simulink model "Combined_DCconv_andMPPT"  (R2023a)
settings: Solver=ode23s  StartTime=0.0  StopTime=0.1  MaxStep=0.0000001  RelTol=1e-4  AbsTol=1e-4
values from neighbouring files (symbols this model uses):
  A = Aoff    [BoostConverterHybrid.m]    (also in PV_Params.mat = 1.3)
  C = [0 1]    [BoostConverterHybrid.m]    (also in boost_converter_sfcnv3.m = u(4); params_dcdc.m = 0.00012878; params_forEVcharge.m = 0.00010675)
  E = u(1)    [boost_converter_sfcnv3.m]    (also in params_forEVcharge.m = 90)
  Isc = 8.61    [PV_Params.mat]    (also in parameterEstimationv2.m = 5.45)
  Ki = 0.05    [PV_Params.mat]
  Kv = -0.32    [PV_Params.mat]
  L = 1    [BoostConverterHybrid.m]    (also in boost_converter_sfcnv3.m = u(3); params_dcdc.m = 0.00035; params_forEVcharge.m = 0.008945)
  Ns = 60    [PV_Params.mat]
  R = 1    [BoostConverterHybrid.m]    (also in boost_converter_sfcnv3.m = u(5); params_dcdc.m = 4.6; params_forEVcharge.m = 48.48)
  Rp = 415    [PV_Params.mat]    (also in battery_params_v2.m = 0.003103; parameterEstimationv2.m = R_p)
  Rs = 0.22    [PV_Params.mat]    (also in battery_params_v2.m = 0.010822; parameterEstimationv2.m = R_s)
  T = 298    [parameterEstimationv2.m]    (also in params_dcdc.m = 1e-05; params_forEVcharge.m = 1e-05)
  Voc = 38.41    [PV_Params.mat]    (also in parameterEstimationv2.m = 43.6)
undefined symbols (not defined in the file or in its folder): sigbuilder_block
libraries: simulink x2, slpidlib x1, SignalEditorBlockLib x1
settings Model: Creator=gabrielcrisan  LastModifiedBy=gabrielcrisan

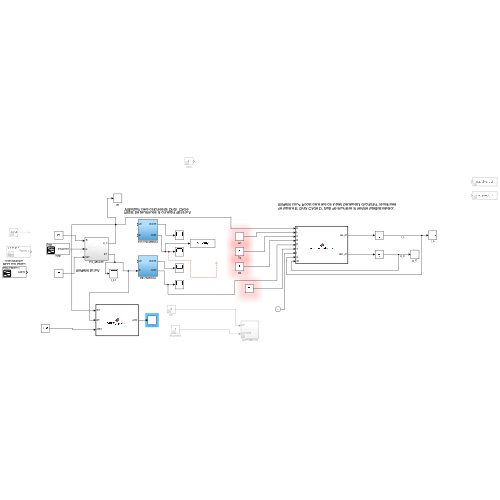
[thumbnail: Simulink's stored preview of the top-level diagram]
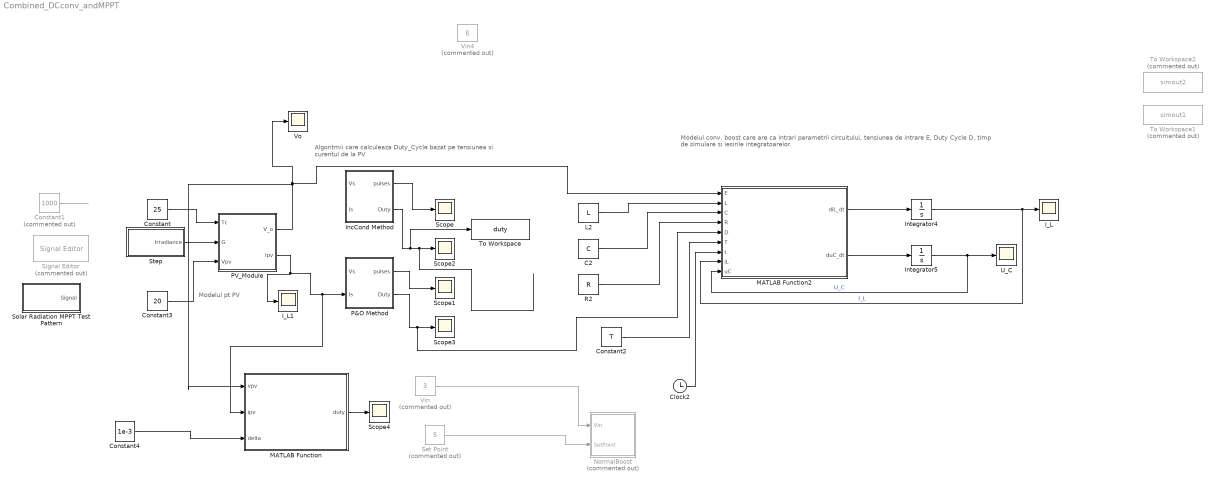
== system Combined_DCconv_andMPPT ==
  note: Modelul pt PV
  note: Algoritmii care calculeaza Duty_Cycle bazat pe tensiunea si curentul de la PV
  note: Modelul conv. boost care are ca intrari parametrii circuitului, tensiunea de intrare E, Duty Cycle D, timp de simulare si iesirile integratoarelor.
  C2 : Constant  Value=C
  Clock2 : Clock
  Constant : Constant  Value=25
  Constant1 : Constant  Commented=on  Value=1000
  Constant2 : Constant  Value=T
  Constant3 : Constant  Value=20
  Constant4 : Constant  Value=1e-3
  I_L : Scope
  I_L1 : Scope
  IncCond Method : Subsystem  VariantControl=MPPT_IncCond
  Integrator4 : Integrator
  Integrator5 : Integrator
  L2 : Constant  Value=L
  MATLAB Function : MATLAB Function  TreatAsAtomicUnit=on
  MATLAB Function2 : MATLAB Function  TreatAsAtomicUnit=on
  NormalBoost : Subsystem  Commented=on
  P&O Method : Subsystem  VariantControl=MPPT_PandO
  PV_Module : Subsystem
  R2 : Constant  Value=R
  Scope{,1..4} (5 alike) : Scope
  Set Point : Constant  Commented=on  Value=5
  Signal Editor : SignalEditorBlockLib/Signal Editor  Commented=on  FileName=untitled.mat  ActiveScenario=Scenario  ActiveSignal=Signal 1  IsBus=off  OutputBusObjectStr=Bus: BusObject  SampleTime=0  Interpolate=off  ZeroCross=off  OutputAfterFinalValue=Setting to zero  Unit=inherit  PreserveSignalName=on  ApplySigPropsToAllScenarios=on
  Solar Radiation MPPT Test Pattern : Subsystem  Tag=STV Subsys  LoadFcn=sigbuilder_block('load',[1935 57 649 359 ]);  StartFcn=sigbuilder_block('start');  StopFcn=sigbuilder_block('stop');  ClipboardFcn=sigbuilder_block('clipboard');  mask(Sigbuilder block){tuvar=[0:10]}
      mask help: Simulink:masks:SigbuilderBlock_MD
      mask init:
      | if ~strcmp(get_param(bdroot(gcbh),'SimulationStatus'),'stopped') tuvar = sigbuilder_block('maskInit'); end
      settings: CopyFcn=sigbuilder_block('copy');  DeleteFcn=sigbuilder_block('delete');  ModelCloseFcn=sigbuilder_block('modelClose');  PreSaveFcn=sigbuilder_block('preSave');  PauseFcn=sigbuilder_block('pause');  ContinueFcn=sigbuilder_block('continue');  NameChangeFcn=sigbuilder_block('namechange');  OpenFcn=sigbuilder_block('open',[330.75 60 648.75 359.25 ]);  CloseFcn=sigbuilder_block('close');
      mask Display: plot(0, 0, 100, 100,[2, 2, 32, 32, 2], [68, 8, 8, 68, 68],[32, 2], [38, 38], [32, 19, 2],[53, 60, 44], [32, 17, 17, 2],[16, 16, 31, 31]);txt = getActiveGroup(gcbh);text(2, 100, txt,'verticalAlignment', 'top');
  Step : Subsystem  Tag=STV Subsys  LoadFcn=sigbuilder_block('load');  StartFcn=sigbuilder_block('start');  StopFcn=sigbuilder_block('stop');  ClipboardFcn=sigbuilder_block('clipboard');  VariantControl=Step  mask(Sigbuilder block){tuvar=[0:10]}
      mask help: Simulink:masks:SigbuilderBlock_MD
      mask init:
      | if ~strcmp(get_param(bdroot(gcbh),'SimulationStatus'),'stopped') tuvar = sigbuilder_block('maskInit'); end
      settings: CopyFcn=sigbuilder_block('copy');  DeleteFcn=sigbuilder_block('delete');  ModelCloseFcn=sigbuilder_block('modelClose');  PreSaveFcn=sigbuilder_block('preSave');  PauseFcn=sigbuilder_block('pause')  ContinueFcn=sigbuilder_block('continue')  NameChangeFcn=sigbuilder_block('namechange');  OpenFcn=sigbuilder_block('open',[1901 151 412 328 ]);  CloseFcn=sigbuilder_block('close');
      mask Display: plot(0, 0, 100, 100,[2, 2, 32, 32, 2], [68, 8, 8, 68, 68],[32, 2], [38, 38], [32, 19, 2],[53, 60, 44], [32, 17, 17, 2],[16, 16, 31, 31]);txt = getActiveGroup(gcbh);text(2, 100, txt,'verticalAlignment', 'top');
  To Workspace : ToWorkspace  VariableName=duty  SaveFormat=Timeseries  SampleTime=-1
  To Workspace1 : ToWorkspace  Commented=on  VariableName=simout1  SaveFormat=Timeseries  SampleTime=-1
  To Workspace2 : ToWorkspace  Commented=on  VariableName=simout2  SaveFormat=Timeseries  SampleTime=-1
  U_C : Scope
  Vin : Constant  Commented=on  Value=3
  Vin4 : Constant  Commented=on  Value=E
  Vo : Scope
  wires:
  C2/1 -> MATLAB Function2/3(C)
  Integrator4/1 -> MATLAB Function2/8(iL), I_L/1  "I_L"
  R2/1 -> MATLAB Function2/4(R)
  MATLAB Function2/1(diL_dt) -> Integrator4/1
  MATLAB Function2/2(duC_dt) -> Integrator5/1
  Clock2/1 -> MATLAB Function2/7(t)
  Constant2/1 -> MATLAB Function2/6(T)
  L2/1 -> MATLAB Function2/2(L)
  P&O Method/2(Duty) -> MATLAB Function2/5(D), Scope3/1
  Integrator5/1 -> U_C/1, MATLAB Function2/9(uC)  "U_C"
  IncCond Method/1(pulses) -> Scope/1
  P&O Method/1(pulses) -> Scope1/1
  IncCond Method/2(Duty) -> Scope2/1, To Workspace/1
  PV_Module/2(Ipv) -> MATLAB Function/2(ipv), P&O Method/2(Is), I_L1/1
  Constant1/1 -> ?
  Constant/1 -> PV_Module/1(Tc)
  PV_Module/1(V_o) -> MATLAB Function/1(vpv), Vo/1, MATLAB Function2/1(E)
  Constant3/1 -> PV_Module/3(Vpv)
  Step/1(Irradiance) -> PV_Module/2(G)
  Set Point/1 -> NormalBoost/2(SetPoint)
  Vin/1 -> NormalBoost/1(Vin)
  Constant4/1 -> MATLAB Function/3(delta)
  MATLAB Function/1(duty) -> Scope4/1

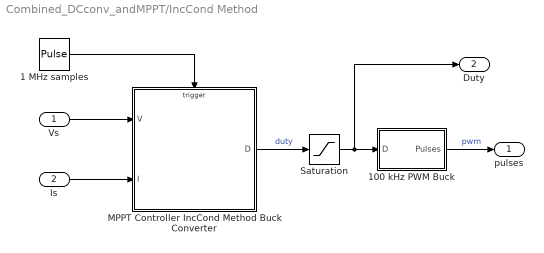
== system Combined_DCconv_andMPPT/IncCond Method ==
  Vs : Inport
  Is : Inport  Port=2
  1 MHz samples : DiscretePulseGenerator  PulseType=Time based  Period=0.000001  PulseWidth=5
  100 kHz PWM Buck : Subsystem  mask{Freq=100000}
      mask prompts: Freq "Frequency (Hz)"
  MPPT Controller IncCond Method Buck Converter : Stateflow chart  TreatAsAtomicUnit=on
  Saturation : Saturate  UpperLimit=1  LowerLimit=0  OutMin=[0]  OutMax=[1]
  pulses : Outport
  Duty : Outport  Port=2
  wires:
  Vs/1 -> MPPT Controller IncCond Method Buck Converter/1(V)
  MPPT Controller IncCond Method Buck Converter/1(D) -> Saturation/1  "duty"
  100 kHz PWM Buck/1(Pulses) -> pulses/1  "pwm"
  1 MHz samples/1 -> MPPT Controller IncCond Method Buck Converter/Trigger
  Saturation/1 -> Duty/1, 100 kHz PWM Buck/1(D)
  Is/1 -> MPPT Controller IncCond Method Buck Converter/2(I)

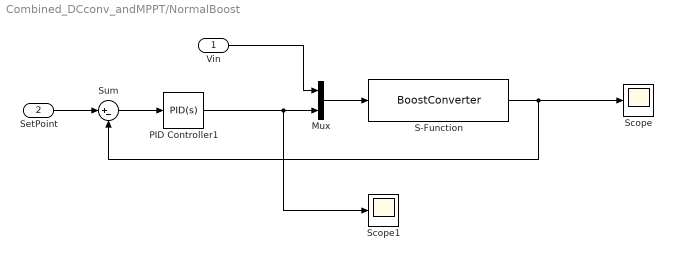
== system Combined_DCconv_andMPPT/NormalBoost ==
  Vin : Inport
  SetPoint : Inport  Port=2
  Mux : Mux  Inputs=2
  PID Controller1 : slpidlib/PID Controller  Controller=PID  Form=Parallel  TimeDomain=Continuous-time  UseExternalTs=off  SampleTime=-1  IntegratorMethod=Forward Euler  FilterMethod=Forward Euler  ControllerParametersSource=internal  P=10  I=0.2  UseKiTs=off  D=0  N=100  UseFilter=on  TunerSelectOption=Transfer Function Based (PID Tuner App)  InitialConditionSource=internal  InitialConditionForIntegrator=0  InitialConditionForFilter=0  DifferentiatorICPrevScaledInput=0  ExternalReset=none  TrackingMode=off  Kt=1  LimitOutput=off  SatLimitsSource=internal  UpperSaturationLimit=inf  LowerSaturationLimit=-inf  LinearizeAsGain=on  AntiWindupMode=none  Kb=1  LimitIntegrator=off  UpperIntegratorSaturationLimit=inf  LowerIntegratorSaturationLimit=-inf  POutMin=[]  POutMax=[]  IOutMin=[]  IOutMax=[]  DOutMin=[]  DOutMax=[]  NOutMin=[]  NOutMax=[]  SumOutMin=[]  SumOutMax=[]  SaturationOutMin=[]  SaturationOutMax=[]  PParamMin=[]  PParamMax=[]  IParamMin=[]  IParamMax=[]  DParamMin=[]  DParamMax=[]  NParamMin=[]  NParamMax=[]  KbParamMin=[]  KbParamMax=[]  KtParamMin=[]  KtParamMax=[]  KbOutMin=[]  KbOutMax=[]  KtOutMin=[]  KtOutMax=[]  IntegratorOutMin=[]  IntegratorOutMax=[]  FilterOutMin=[]  FilterOutMax=[]  SumI1OutMin=[]  SumI1OutMax=[]  SumI2OutMin=[]  SumI2OutMax=[]  SumI3OutMin=[]  SumI3OutMax=[]  SumI4OutMin=[]  SumI4OutMax=[]  SumDOutMin=[]  SumDOutMax=[]  DifferentiatorOutMin=[]  DifferentiatorOutMax=[]  FilterDiffOutCoefMin=[]  FilterDiffOutCoefMax=[]  ReciprocalOutMin=[]  ReciprocalOutMax=[]  SumDenOutMin=[]  SumDenOutMax=[]  SumNumOutMin=[]  SumNumOutMax=[]  DivideOutMin=[]  DivideOutMax=[]  UdiffTsProdOutMin=[]  UdiffTsProdOutMax=[]  NTsProdOutMin=[]  NTsProdOutMax=[]  UintegralTsProdOutMin=[]  UintegralTsProdOutMax=[]  UngainTsProdOutMin=[]  UngainTsProdOutMax=[]  ClampingZeroOutDataTypeStr=Inherit: Inherit via back propagation  ClampingZeroOutMin=[]  ClampingZeroOutMax=[]  FilterDenConstantOutDataTypeStr=Inherit: Inherit via back propagation  FilterDenConstantOutMin=[]  FilterDenConstantOutMax=[]  PCopyOutDataTypeStr=Inherit: Inherit via back propagation  PCopyOutMin=[]  PCopyOutMax=[]  NCopyOutDataTypeStr=Inherit: Inherit via back propagation  NCopyOutMin=[]  NCopyOutMax=[]  IntegratorContinuousStateAttributes=''  IntegratorStateMustResolveToSignalObject=off  IntegratorRTWStateStorageClass=Auto  FilterContinuousStateAttributes=''  FilterStateMustResolveToSignalObject=off  FilterRTWStateStorageClass=Auto  ParallelPVariant=InternalParameters  IdealPVariant=Disabled  IVariant=InternalParameters  DVariant=InternalParameters  IntegratorVariant=Continuous  SatVariant=Disabled  AWVariant=Passthrough  PCopyVariant=Disabled  TRVariant=Disabled  FdbkBlocksVariant=Forward  IdealPFdbkVariant=Disabled  SatFdbkVariant=Disabled  DerivativeFilterVariant=ContFilter  NVariant=InternalParameters  NCopyVariant=Disabled  FilterICVariant=InternalICsFilter  IntegratorICVariant=InternalICs  ExternalResetVariant=Disabled  TRSumVariant=Passthrough  SumFdbkVariant=Disabled  SumVariant=Sum_PID  TsampFilterVariant=InternalTs  TsampNgainVariant=Passthrough  TsampIntegralVariant=Disabled_SignalSpec  ExternalSaturationOutDataTypeStr=Inherit: Same as second input
  S-Function : S-Function  FunctionName=BoostConverter  SFunctionDeploymentMode=off  EnableBusSupport=off
  Scope : Scope
  Scope1 : Scope
  Sum : Sum  Inputs=|+-
  wires:
  Mux/1 -> S-Function/1
  Sum/1 -> PID Controller1/1
  Vin/1 -> Mux/1
  S-Function/1 -> Sum/2, Scope/1
  SetPoint/1 -> Sum/1
  PID Controller1/1 -> Scope1/1, Mux/2

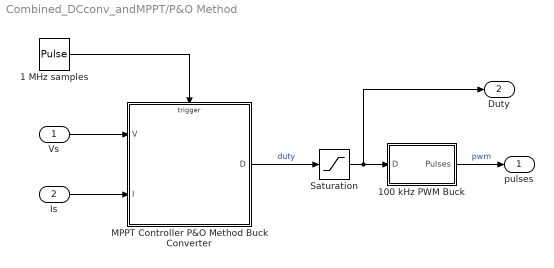
== system Combined_DCconv_andMPPT/P&O Method ==
  Vs : Inport
  Is : Inport  Port=2
  1 MHz samples : DiscretePulseGenerator  PulseType=Time based  Period=0.000001  PulseWidth=5
  100 kHz PWM Buck : Subsystem  mask{Freq=100000}
      mask prompts: Freq "Frequency (Hz)"
  MPPT Controller P&O Method Buck Converter : Stateflow chart  TreatAsAtomicUnit=on
  Saturation : Saturate  UpperLimit=1  LowerLimit=0  OutMin=[0]  OutMax=[1]
  pulses : Outport
  Duty : Outport  Port=2
  wires:
  100 kHz PWM Buck/1(Pulses) -> pulses/1  "pwm"
  Is/1 -> MPPT Controller P&O Method Buck Converter/2(I)
  Vs/1 -> MPPT Controller P&O Method Buck Converter/1(V)
  Saturation/1 -> Duty/1, 100 kHz PWM Buck/1(D)
  1 MHz samples/1 -> MPPT Controller P&O Method Buck Converter/Trigger
  MPPT Controller P&O Method Buck Converter/1(D) -> Saturation/1  "duty"

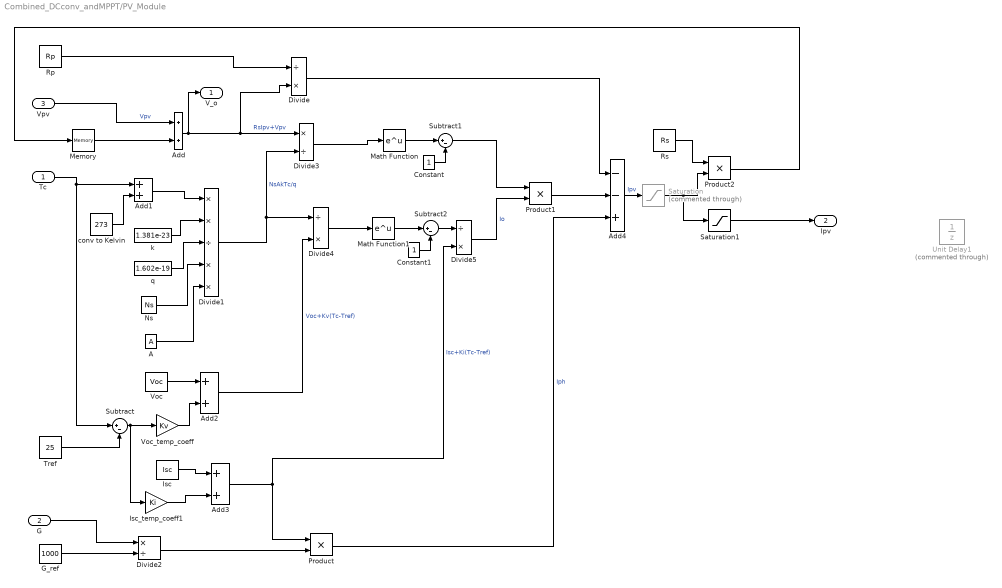
== system Combined_DCconv_andMPPT/PV_Module ==
  Tc : Inport
  G : Inport  Port=2
  Vpv : Inport  Port=3
  A : Constant  Value=A
  Add{,1..3} (4 alike) : Sum
  Add4 : Sum  Inputs=--+
  Constant : Constant
  Constant1 : Constant
  Divide : Product  Inputs=/*
  Divide1 : Product  Inputs=**/**
  Divide2 : Product  Inputs=*/
  Divide3 : Product  Inputs=*/
  Divide4 : Product  Inputs=/*
  Divide5 : Product  Inputs=/*
  G_ref : Constant  Value=1000
  Isc : Constant  Value=Isc
  Isc_temp_coeff1 : Gain  Gain=Ki
  Math Function : Math
  Math Function1 : Math
  Memory : Memory  InheritSampleTime=on
  Ns : Constant  Value=Ns
  Product : Product
  Product1 : Product
  Product2 : Product
  Rp : Constant  Value=Rp
  Rs : Constant  Value=Rs
  Saturation : Saturate  Commented=through  UpperLimit=inf  LowerLimit=0
  Saturation1 : Saturate  UpperLimit=inf  LowerLimit=0
  Subtract : Sum  Inputs=|+-
  Subtract1 : Sum  Inputs=|+-
  Subtract2 : Sum  Inputs=|+-
  Tref : Constant  Value=25
  Unit Delay1 : UnitDelay  Commented=through  SampleTime=-1  HasFrameUpgradeWarning=on
  Voc : Constant  Value=Voc
  Voc_temp_coeff : Gain  Gain=Kv
  conv to Kelvin : Constant  Value=273
  k : Constant  Value=1.381e-23
  q : Constant  Value=1.602e-19
  V_o : Outport
  Ipv : Outport  Port=2
  wires:
  Add1/1 -> Divide1/1
  Product/1 -> Add4/3  "Iph"
  k/1 -> Divide1/2
  Vpv/1 -> Add/1  "Vpv"
  Constant/1 -> Subtract1/2
  Add/1 -> V_o/1, Divide/2, Divide3/1  "RsIpv+Vpv"
  Divide5/1 -> Product1/2  "Io"
  Tc/1 -> Subtract/1, Add1/1
  Add3/1 -> Divide5/2, Product/1  "Isc+Ki(Tc-Tref)"
  Constant1/1 -> Subtract2/2
  Subtract1/1 -> Product1/1
  Divide4/1 -> Math Function1/1
  Divide1/1 -> Divide4/1, Divide3/2  "NsAkTc/q"
  Math Function/1 -> Subtract1/1
  q/1 -> Divide1/3
  Isc/1 -> Add3/1
  Voc_temp_coeff/1 -> Add2/2
  A/1 -> Divide1/5
  Tref/1 -> Subtract/2
  G_ref/1 -> Divide2/2
  Add4/1 -> Saturation/1  "Ipv"
  conv to Kelvin/1 -> Add1/2
  G/1 -> Divide2/1
  Subtract/1 -> Isc_temp_coeff1/1, Voc_temp_coeff/1
  Rp/1 -> Divide/1
  Ns/1 -> Divide1/4
  Isc_temp_coeff1/1 -> Add3/2
  Voc/1 -> Add2/1
  Math Function1/1 -> Subtract2/1
  Add2/1 -> Divide4/2  "Voc+Kv(Tc-Tref)"
  Subtract2/1 -> Divide5/1
  Rs/1 -> Product2/1
  Divide2/1 -> Product/2
  Divide3/1 -> Math Function/1
  Memory/1 -> Add/2
  Saturation/1 -> Saturation1/1, Product2/2
  Product2/1 -> Memory/1
  Divide/1 -> Add4/1
  Product1/1 -> Add4/2
  Saturation1/1 -> Ipv/1

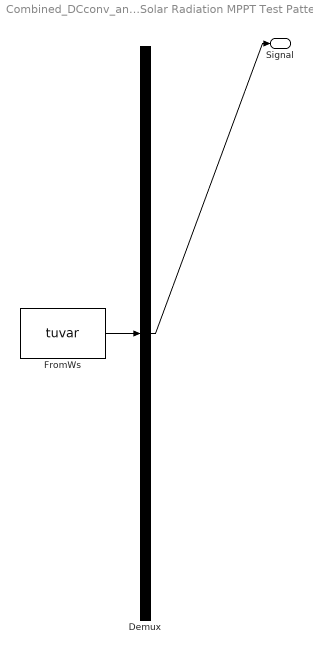
== system Combined_DCconv_andMPPT/Solar Radiation MPPT Test Pattern ==
  Demux : Demux  Tag=STV Demux  Outputs=1
      settings: DisplayOption=none
  FromWs : FromWorkspace  Tag=STV FromWs  VariableName=tuvar
      SigBuilderData=|
      | common.afterFinalStr = 'Extrapolate'
      | common.sampleTime = 0
      | dataSet.timeRange = [0 60]
      | dataSet.name = 'Test Pattern 1'
      | sbobj.Groups.Name = 'Test Pattern 1'
      | sbobj.Groups.Signals.Name = 'Signal'
      | sbobj.Groups.Signals.XData = [0 2 2 4 4 6 6 8 8 10 10 12 12 14 14 16 16 18 18 20 20 22 22 51.6 51.6 57.8 60]
      | sbobj.Groups.Signals.YData = [100 100 200 200 300 300 400 400 500 500 600 600 700 700 800 800 900 900 1000 1000 100 100 1000 1000 195 195 195]
      | sbobj.Groups.TimeRange = [0 60]
  Signal : Outport  Tag=STV Outport  VectorParamsAs1DForOutWhenUnconnected=off
  wires:
  Demux/1 -> Signal/1
  FromWs/1 -> Demux/1

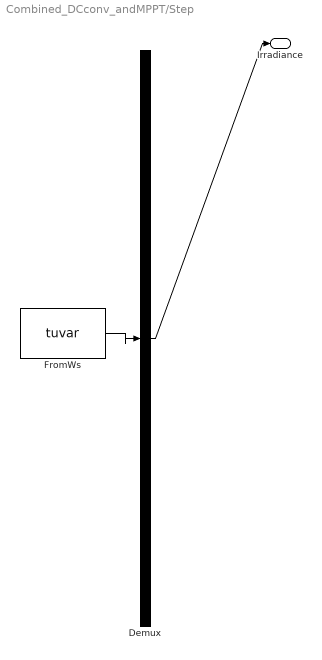
== system Combined_DCconv_andMPPT/Step ==
  Demux : Demux  Tag=STV Demux  Outputs=1
      settings: DisplayOption=none
  FromWs : FromWorkspace  Tag=STV FromWs  VariableName=tuvar
      SigBuilderData=|
      | common.afterFinalStr = 'Extrapolate'
      | common.sampleTime = 0
      | dataSet.timeRange = [0 0.1]
      | dataSet.name = 'Step'
      | sbobj.Groups.Name = 'Step'
      | sbobj.Groups.Signals.Name = 'Irradiance'
      | sbobj.Groups.Signals.XData = [0 0.02 0.02 0.04 0.04 0.06 0.06 0.08 0.08 0.1]
      | sbobj.Groups.Signals.YData = [800 800 600 600 1000 1000 800 800 600 600]
      | sbobj.Groups.TimeRange = [0 0.1]
  Irradiance : Outport  Tag=STV Outport
  wires:
  Demux/1 -> Irradiance/1
  FromWs/1 -> Demux/1

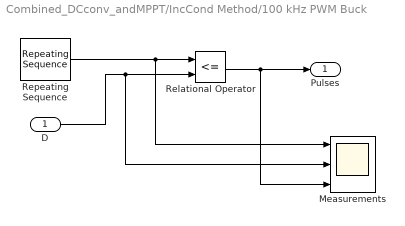
== system Combined_DCconv_andMPPT/IncCond Method/100 kHz PWM Buck ==
  D : Inport
  Measurements : Scope  NumInputPorts=3
  Relational Operator : RelationalOperator  Operator=<=  OutDataTypeStr=boolean  ZeroCross=off  InputSameDT=off
  Repeating Sequence : simulink/Sources/Repeating Sequence  rep_seq_t="[0  1/Freq]"  rep_seq_y=[0 1]
  Pulses : Outport
  wires:
  D/1 -> Relational Operator/2, Measurements/2
  Relational Operator/1 -> Pulses/1, Measurements/3
  Repeating Sequence/1 -> Relational Operator/1, Measurements/1

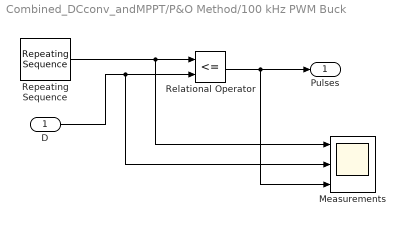
== system Combined_DCconv_andMPPT/P&O Method/100 kHz PWM Buck ==
  D : Inport
  Measurements : Scope  NumInputPorts=3
  Relational Operator : RelationalOperator  Operator=<=  OutDataTypeStr=boolean  ZeroCross=off  InputSameDT=off
  Repeating Sequence : simulink/Sources/Repeating Sequence  rep_seq_t="[0  1/Freq]"  rep_seq_y=[0 1]
  Pulses : Outport
  wires:
  Repeating Sequence/1 -> Measurements/1, Relational Operator/1
  Relational Operator/1 -> Measurements/3, Pulses/1
  D/1 -> Measurements/2, Relational Operator/2

== stateflow chart Combined_DCconv_andMPPT/IncCond Method/MPPT Controller IncCond Method Buck Converter ==
  state AVERAGE100SAMPLES
    entry:
    Vsum = 0; Isum = 0; k = 0;
    during:
    Vsum = Vsum + V;
    Isum = Isum + I; k++;
    exit:
    Vavg = Vsum/k;
    Iavg = Isum/k;
  state SAMPLEandCALCULATE
    entry:
    deltaV = Vavg - Vprev;
    deltaI = Iavg - Iprev;
    d = D;
  state DECREMENT
    entry:
    d = d - deltad;
  state INCREMENT
    entry:
    d = d + deltad;
  state RETURN
    entry:
    Vprev = Vavg;
    Iprev = Iavg;
    D = d;
  RETURN -> AVERAGE100SAMPLES
  (default) -> AVERAGE100SAMPLES
  AVERAGE100SAMPLES -> SAMPLEandCALCULATE : after(100,clk)
  SAMPLEandCALCULATE -> (junction 16) [order 1] : [deltaV~=0]
  SAMPLEandCALCULATE -> (junction 17) [order 2] : [deltaV==0]
  (junction 17) -> INCREMENT [order 1] : [deltaI < 0]
  (junction 17) -> RETURN [order 3] : [deltaI == 0]
  (junction 16) -> RETURN [order 3] : [deltaI/deltaV == -Iavg/Vavg]
  (junction 16) -> DECREMENT [order 1] : [deltaI/deltaV > -Iavg/Vavg]
  (junction 17) -> DECREMENT [order 2] : [deltaI > 0]
  (junction 16) -> INCREMENT [order 2] : [deltaI/deltaV < -Iavg/Vavg]
  DECREMENT -> RETURN
  INCREMENT -> RETURN
  data: V input; I input; D output double =0.7; k local double; Iavg local double; Iprev local double; Isum local double; Vavg local double; Vprev local double; Vsum local double; d local double; deltaI local double; deltaV local double; deltad local double =8e-3
  events: clk input RISING_EDGE_EVENT

== matlab function Combined_DCconv_andMPPT/MATLAB Function ==
  settings: updateMethod=DISCRETE
  data: vpv input; duty output; ipv input; delta input
% MPPT
function duty = MPPT_algorithm(vpv,ipv,delta)
% Incremental Conductance MPPT algorithm 
duty_init = 0.5;
% Min and max value are used to limit duty between 0 and 1
duty_min=0;
duty_max=1;

persistent Vold Pold duty_old;
% Persistent variable type can store the data
% We need the old data by obtaining difference between old and new value
if isempty(Vold)
    Vold=0;
    Pold=0;
    duty_old=duty_init;
end
P= vpv*ipv; % power
dV= vpv - Vold; % difference between old and new voltage
dP= P - Pold;% difference between old and new power

% The algorithm in below search the dP/dV=0
% If the derivative equal to zero
% duty will not change if old and new power not equal &
% pv voltage bigger than 30V the algorithm will work
if dP ~= 0 && vpv>30
    if dP < 0
        if dV < 0
            duty = duty_old - delta;
        else
            duty = duty_old + delta;
        end
    else
        if dV < 0
            duty = duty_old + delta;
        else
            duty = duty_old - delta;
        end
    end
else
    duty = duty_old;
end

%If limits the duty between min and max
if duty >= duty_max
    duty=duty_max;
elseif duty<duty_min
    duty=duty_min;
end

% Stored data
duty_old=duty;
Vold=vpv;
Pold=P;

== matlab function Combined_DCconv_andMPPT/MATLAB Function2 ==
  settings: updateMethod=DISCRETE
  data: E input; L input; C input; R input; D input; T input; t input; diL_dt output; iL input; uC input; duC_dt output
function [diL_dt, duC_dt] = boost_converter_func(E, L, C, R, D, T, t, iL, uC)
    
    persistent t_last_switch interval

    if isempty(t_last_switch)
        t_last_switch = 0;
        interval = 1;  % Start with switch on
    end

    t_since_switch = t - t_last_switch;

    if interval == 1 && t_since_switch >= D * T
        interval = 2;  % Switch off
        t_last_switch = t;
    elseif interval == 2 && t_since_switch >= (1 - D) * T
        interval = 3;  % Enter discontinuous mode (if applicable)
        t_last_switch = t;
    elseif interval == 3 && t_since_switch >= (1 - D) * T
        interval = 1;  % Switch on again
        t_last_switch = t;
    end

    % Initialize outputs
    diL_dt = 0;
    duC_dt = 0;

    switch interval
        case 1  % Switch is on, Diode is off
            diL_dt = E / L;
            duC_dt = -uC / (R * C);
        case 2  % Switch is off, Diode is on
            diL_dt = (E - uC) / L;
            duC_dt = (iL - uC / R) / C;
        case 3  % Discontinuous mode, both switch and diode off
            diL_dt = 0;
            duC_dt = -uC / (R * C);
    end
end

== stateflow chart Combined_DCconv_andMPPT/P&O Method/MPPT Controller P&O Method Buck Converter ==
  state AVERAGE100SAMPLES
    entry:
    P = V*I; Psum = 0; Vsum = 0; k = 0;
    during:
    Psum = Psum +P; Vsum = Vsum + V; k++;
    exit:
    Pavg = Psum/k; Vavg = Vsum/k;
  state SAMPLEandCALCULATE
    entry:
    deltaP = Pavg - Pprev;
    deltaV = Vavg - Vprev;
    d = D;
  state DECREMENT
    entry:
    d = d - deltad;
  state INCREMENT
    entry:
    d = d + deltad;
  state RETURN
    entry:
    Pprev = Pavg; Vprev = Vavg; D = d;
  RETURN -> AVERAGE100SAMPLES
  (default) -> AVERAGE100SAMPLES
  AVERAGE100SAMPLES -> SAMPLEandCALCULATE : after(100,clk)
  SAMPLEandCALCULATE -> RETURN [order 1] : [deltaP==0]
  SAMPLEandCALCULATE -> (junction 138) [order 3] : [deltaP < 0]
  SAMPLEandCALCULATE -> (junction 139) [order 2] : [deltaP >0]
  (junction 139) -> INCREMENT [order 1] : [deltaV < 0]
  (junction 138) -> DECREMENT [order 2] : [deltaV < 0]
  (junction 139) -> DECREMENT [order 2] : [deltaV > 0]
  (junction 138) -> INCREMENT [order 1] : [deltaV > 0]
  DECREMENT -> RETURN
  INCREMENT -> RETURN
  data: V input; I input; D output double =0.7; k local double; Vavg local double; Vprev local double; Vsum local double; d local double; deltaV local double; deltad local double =8e-3; P local double; Pavg local double; Pprev local double; Psum local double; deltaP local double
  events: clk input RISING_EDGE_EVENT
